simulink model "NACA_0021"  (R2023b)
settings: Solver=VariableStepAuto  StartTime=0.0  StopTime=12  RelTol=1e-3
InitFcn:
  | init
settings Model: Creator=HQ03  LastModifiedBy=dzxion_microsoft
settings OptimizationCC: ReuseModelBlockBuffer=off

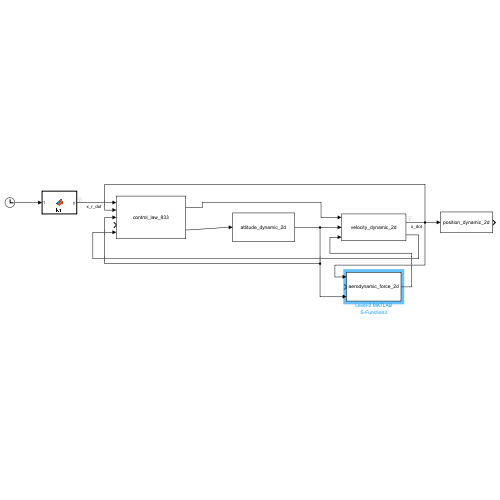
[thumbnail: Simulink's stored preview of the top-level diagram]
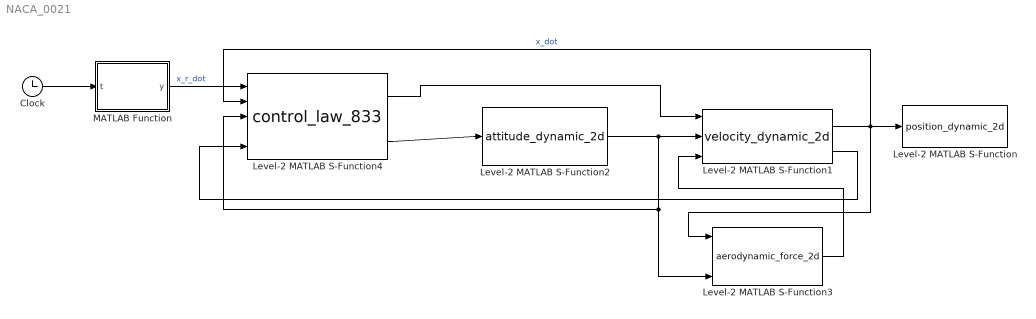
== system NACA_0021 ==
  Clock : Clock
  Level-2 MATLAB S-Function : M-S-Function  FunctionName=position_dynamic_2d  Parameters=pa
  Level-2 MATLAB S-Function1 : M-S-Function  FunctionName=velocity_dynamic_2d  Parameters=pa
  Level-2 MATLAB S-Function2 : M-S-Function  FunctionName=attitude_dynamic_2d
  Level-2 MATLAB S-Function3 : M-S-Function  FunctionName=aerodynamic_force_2d  Parameters=pa
  Level-2 MATLAB S-Function4 : M-S-Function  FunctionName=control_law_833  Parameters=pa
  MATLAB Function : MATLAB Function  TreatAsAtomicUnit=on
  wires:
  Level-2 MATLAB S-Function1/1 -> Level-2 MATLAB S-Function4/2, Level-2 MATLAB S-Function3/1, Level-2 MATLAB S-Function/1  "x_dot"
  Level-2 MATLAB S-Function2/1 -> Level-2 MATLAB S-Function4/3, Level-2 MATLAB S-Function3/3, Level-2 MATLAB S-Function1/2
  Level-2 MATLAB S-Function3/1 -> Level-2 MATLAB S-Function1/3
  Level-2 MATLAB S-Function1/2 -> Level-2 MATLAB S-Function4/5
  Level-2 MATLAB S-Function4/1 -> Level-2 MATLAB S-Function1/1
  Level-2 MATLAB S-Function4/2 -> Level-2 MATLAB S-Function2/1
  Clock/1 -> MATLAB Function/1(t)
  MATLAB Function/1(y) -> Level-2 MATLAB S-Function4/1  "x_r_dot"

== matlab function NACA_0021/MATLAB Function ==
  data: t input; y output
function y = fcn(t)

if t<=10
    x_r_dot = [0;2*t];
else
    x_r_dot = [0;20];
end

y = x_r_dot;
